simulink model "Flowchart9"  (Simulink 8.7)
settings: Solver=FixedStepDiscrete  StartTime=0.0  StopTime=10.0  RelTol=1e-3
settings Model: Creator=scaife  LastModifiedBy=bourbouh  ExtModeAutoUpdateStatusClock=off
settings DataIOCC: SignalLoggingSaveFormat=ModelDataLogs
settings OptimizationCC: InitFltsAndDblsToZero=on
settings DebuggingCC: SaveWithParameterizedLinksMsg=none  SignalResolutionControl=TryResolveAllWithWarning  SolverPrmCheckMsg=warning  MultiTaskDSMMsg=warning  MultiTaskCondExecSysMsg=none  StrictBusMsg=None
settings SFSimCC: SimParseCustomCode=off
settings GRTTargetCC: TargetFcnLib=ansi_tfl_tmw.mat  GeneratePreprocessorConditionals=Use local settings  CombineOutputUpdateFcns=off  GRTInterface=on

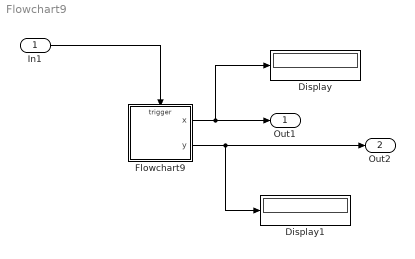
== system Flowchart9 ==
  In1 : Inport
  Display : Display
  Display1 : Display
  Flowchart9 : Stateflow chart  TreatAsAtomicUnit=on
  Out1 : Outport
  Out2 : Outport  Port=2
  wires:
  Flowchart9/1(x) -> Display/1, Out1/1
  Flowchart9/2(y) -> Out2/1, Display1/1
  In1/1 -> Flowchart9/Trigger

== stateflow chart Flowchart9 ==
  state TOP [parallel]
    settings: executionOrder=1
    state A
      A -> (junction 6) [order 1] : {x++}
    state B
      B -> (junction 8) [order 1] : {y++}
    (default) -> A
    A -> B [order 1] : E
    B -> A [order 1] : E
  data: x output int32; y output int32
  events: E input EITHER_EDGE_EVENT
